simulink model "lab8_5"  (R2018b)
settings: Solver=FixedStepDiscrete  StartTime=0.0  StopTime=50000  FixedStep=1  RelTol=1e-3
libraries: hdlsllib x6, simulink x3
settings Model: Creator=mllax8  LastModifiedBy=mllax8

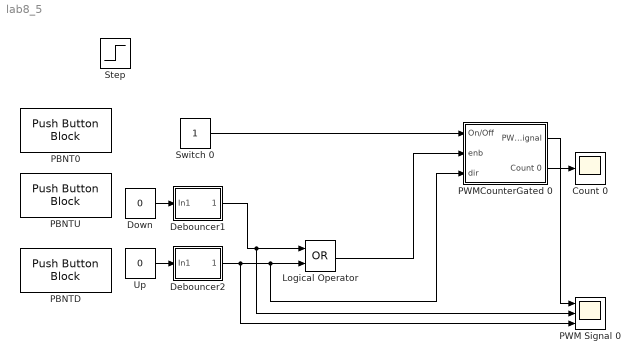
== system lab8_5 ==
  Count 0 : Scope
  Debouncer1 : Subsystem
  Debouncer2 : Subsystem
  Down : Constant  Value=0
  Logical Operator : Logic  Operator=OR  AllPortsSameDT=off  OutDataTypeStr=boolean
  PBNT0 : PushButtonBlock  WebBlockId=175
  PBNTD : PushButtonBlock  WebBlockId=8
  PBNTU : PushButtonBlock  WebBlockId=9
  PWM Signal 0 : Scope  NumInputPorts=3
  PWMCounterGated 0 : Subsystem
  Step : Step  Time=12500  SampleTime=0
  Switch 0 : Constant
  Up : Constant  Value=0
  wires:
  Debouncer1/1(Out1) -> PWM Signal 0/2, Logical Operator/1
  Debouncer2/1(Out1) -> PWM Signal 0/3, PWMCounterGated 0/3(dir), Logical Operator/2
  Switch 0/1 -> PWMCounterGated 0/1(On/Off)
  Logical Operator/1 -> PWMCounterGated 0/2(enb)
  PWMCounterGated 0/1(PWM Signal) -> PWM Signal 0/1
  PWMCounterGated 0/2(Count 0) -> Count 0/1
  Up/1 -> Debouncer2/1(In1)
  Down/1 -> Debouncer1/1(In1)

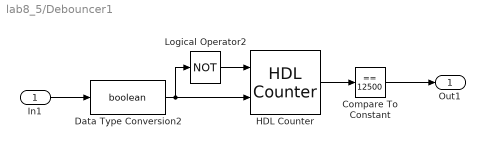
== system lab8_5/Debouncer1 ==
  In1 : Inport
  Compare To Constant : simulink/Logic and Bit Operations/Compare To Constant  relop===  const=12500  OutDataTypeStr=boolean
  Data Type Conversion2 : DataTypeConversion  OutDataTypeStr=boolean
  "HDL Counter " : hdlsllib/Sources/HDL Counter  CountType=Count limited  CountInit=0  CountStep=1  CountMax=50000  CountFromType=Initial value  CountFrom=0  CountResetPort=on  CountLoadPort=off  CountEnbPort=on  CountDirPort=off  CountDataType=Unsigned  CountWordLen=18  CountFracLen=0  CountSampTime=1
      settings: SourceProductBaseCode=HD
  Logical Operator2 : Logic  Operator=NOT  AllPortsSameDT=off  OutDataTypeStr=boolean
  Out1 : Outport
  wires:
  "HDL Counter "/1 -> Compare To Constant/1
  In1/1 -> Data Type Conversion2/1
  Logical Operator2/1 -> "HDL Counter "/1
  Compare To Constant/1 -> Out1/1
  Data Type Conversion2/1 -> "HDL Counter "/2, Logical Operator2/1

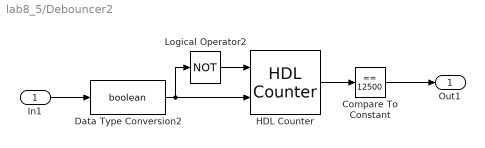
== system lab8_5/Debouncer2 ==
  In1 : Inport
  Compare To Constant : simulink/Logic and Bit Operations/Compare To Constant  relop===  const=12500  OutDataTypeStr=boolean
  Data Type Conversion2 : DataTypeConversion  OutDataTypeStr=boolean
  "HDL Counter " : hdlsllib/Sources/HDL Counter  CountType=Count limited  CountInit=0  CountStep=1  CountMax=50000  CountFromType=Initial value  CountFrom=0  CountResetPort=on  CountLoadPort=off  CountEnbPort=on  CountDirPort=off  CountDataType=Unsigned  CountWordLen=18  CountFracLen=0  CountSampTime=1
      settings: SourceProductBaseCode=HD
  Logical Operator2 : Logic  Operator=NOT  AllPortsSameDT=off  OutDataTypeStr=boolean
  Out1 : Outport
  wires:
  "HDL Counter "/1 -> Compare To Constant/1
  In1/1 -> Data Type Conversion2/1
  Logical Operator2/1 -> "HDL Counter "/1
  Compare To Constant/1 -> Out1/1
  Data Type Conversion2/1 -> "HDL Counter "/2, Logical Operator2/1

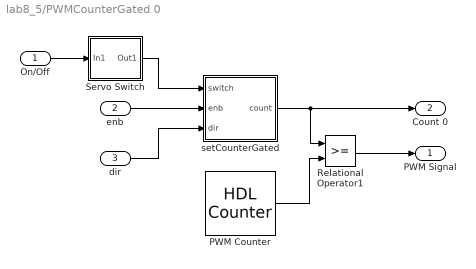
== system lab8_5/PWMCounterGated 0 ==
  On/Off : Inport
  enb : Inport  Port=2
  dir : Inport  Port=3
  "PWM Counter " : hdlsllib/Sources/HDL Counter  CountType=Count limited  CountInit=0  CountStep=1  CountMax=1000  CountFromType=Initial value  CountFrom=0  CountResetPort=off  CountLoadPort=off  CountEnbPort=off  CountDirPort=off  CountDataType=Unsigned  CountWordLen=18  CountFracLen=0  CountSampTime=1
      settings: SourceProductBaseCode=HD
  Relational Operator1 : RelationalOperator  OutDataTypeStr=boolean  RndMeth=Simplest
  Servo Switch : Subsystem
  setCounterGated : Subsystem
  PWM Signal : Outport
  Count 0 : Outport  Port=2
  wires:
  On/Off/1 -> Servo Switch/1(In1)
  setCounterGated/1(count) -> Count 0/1, Relational Operator1/1
  "PWM Counter "/1 -> Relational Operator1/2
  dir/1 -> setCounterGated/3(dir)
  enb/1 -> setCounterGated/2(enb)
  Relational Operator1/1 -> PWM Signal/1
  Servo Switch/1(Out1) -> setCounterGated/1(switch)

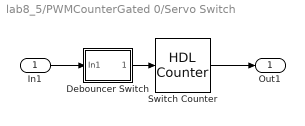
== system lab8_5/PWMCounterGated 0/Servo Switch ==
  In1 : Inport
  Debouncer Switch : Subsystem
  Switch Counter : hdlsllib/Sources/HDL Counter  CountType=Free running  CountInit=0  CountStep=1  CountMax=1  CountFromType=Initial value  CountFrom=0  CountResetPort=off  CountLoadPort=off  CountEnbPort=on  CountDirPort=off  CountDataType=Unsigned  CountWordLen=1  CountFracLen=0  CountSampTime=1
      settings: SourceProductBaseCode=HD
  Out1 : Outport
  wires:
  Debouncer Switch/1(Out1) -> Switch Counter/1
  In1/1 -> Debouncer Switch/1(In1)
  Switch Counter/1 -> Out1/1

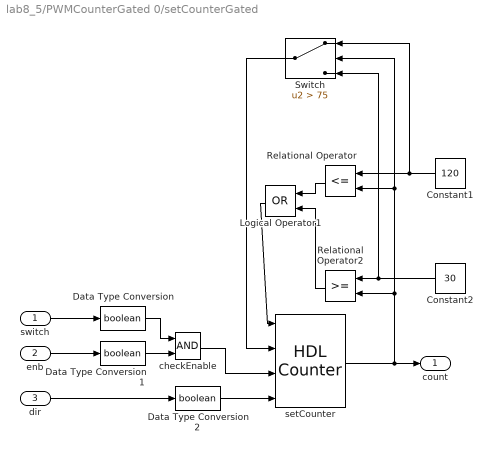
== system lab8_5/PWMCounterGated 0/setCounterGated ==
  switch : Inport
  enb : Inport  Port=2
  dir : Inport  Port=3
  Constant1 : Constant  Value=120  OutDataTypeStr=double  SampleTime=1
  Constant2 : Constant  Value=30  OutDataTypeStr=double  SampleTime=1
  Data Type Conversion : DataTypeConversion  OutDataTypeStr=boolean
  Data Type Conversion1 : DataTypeConversion  OutDataTypeStr=boolean
  Data Type Conversion2 : DataTypeConversion  OutDataTypeStr=boolean
  Logical Operator1 : Logic  Operator=OR  AllPortsSameDT=off  OutDataTypeStr=boolean
  Relational Operator : RelationalOperator  Operator=<=  OutDataTypeStr=boolean  RndMeth=Simplest
  Relational Operator2 : RelationalOperator  OutDataTypeStr=boolean  RndMeth=Simplest
  Switch : Switch  Criteria=u2 > Threshold  Threshold=75  OutDataTypeStr=int16
      settings: LockScale=on
  checkEnable : Logic  AllPortsSameDT=off  OutDataTypeStr=boolean
  setCounter : hdlsllib/Sources/HDL Counter  CountType=Free running  CountInit=75  CountStep=6  CountMax=120  CountFromType=Initial value  CountFrom=75  CountResetPort=off  CountLoadPort=on  CountEnbPort=on  CountDirPort=on  CountDataType=Signed  CountWordLen=16  CountFracLen=0  CountSampTime=1
      settings: SourceProductBaseCode=HD
  count : Outport
  wires:
  switch/1 -> Data Type Conversion/1
  Switch/1 -> setCounter/2
  Data Type Conversion/1 -> checkEnable/1
  Logical Operator1/1 -> setCounter/1
  Data Type Conversion2/1 -> setCounter/4
  Constant1/1 -> Switch/1, Relational Operator/1
  enb/1 -> Data Type Conversion1/1
  Data Type Conversion1/1 -> checkEnable/2
  Relational Operator2/1 -> Logical Operator1/2
  dir/1 -> Data Type Conversion2/1
  Relational Operator/1 -> Logical Operator1/1
  Constant2/1 -> Switch/3, Relational Operator2/1
  checkEnable/1 -> setCounter/3
  setCounter/1 -> count/1, Relational Operator2/2, Relational Operator/2, Switch/2

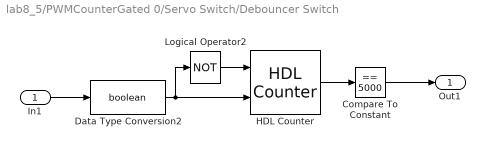
== system lab8_5/PWMCounterGated 0/Servo Switch/Debouncer Switch ==
  In1 : Inport
  Compare To Constant : simulink/Logic and Bit Operations/Compare To Constant  relop===  const=5000  OutDataTypeStr=boolean
  Data Type Conversion2 : DataTypeConversion  OutDataTypeStr=boolean
  "HDL Counter " : hdlsllib/Sources/HDL Counter  CountType=Count limited  CountInit=0  CountStep=1  CountMax=50000  CountFromType=Initial value  CountFrom=0  CountResetPort=on  CountLoadPort=off  CountEnbPort=on  CountDirPort=off  CountDataType=Unsigned  CountWordLen=18  CountFracLen=0  CountSampTime=1
      settings: SourceProductBaseCode=HD
  Logical Operator2 : Logic  Operator=NOT  AllPortsSameDT=off  OutDataTypeStr=boolean
  Out1 : Outport
  wires:
  "HDL Counter "/1 -> Compare To Constant/1
  In1/1 -> Data Type Conversion2/1
  Logical Operator2/1 -> "HDL Counter "/1
  Compare To Constant/1 -> Out1/1
  Data Type Conversion2/1 -> "HDL Counter "/2, Logical Operator2/1
